simulink model "AGTF30SysDyn_PExPIn"  (R2021b)
settings: Solver=ode4  StartTime=0.0  StopTime=MWS.In.tend  FixedStep=MWS.In.Ts  RelTol=1e-3  EnableMultiTasking=on
model workspace: external: MAT-File (data not in the file)
values from neighbouring files (symbols this model uses):
  MWS = setup_initialize(MWS,startPt,SSsolverSP)    [Setup_Simulation.m]    (also in run_AGTF30e_script.m = Setup_Simulation(inputMethod,MWS.In,filename,Mdl,SSsolverSP,)
undefined symbols (not defined in the file or in its folder): DiscIntNeverNeededParam
libraries: Lib_Solve_ModelSource_TMATS x28, Lib_Cntrl_FirstOrderSensor_TMATS x19, simulink x12, Lib_Cntrl_FirstOrderActuator_TMATS x2, Lib_Cntrl_LimitSelect_TMATS x2, Lib_Solve_OuterLoopIntegrator_TMATS x2, Lib_Cntrl_CorrectedSpeed_TMATS x1, Lib_Solve_IterNRSolverJC_TMATS x1
(part 4 of 6)

== system AGTF30SysDyn_PExPIn/Control System/Wf Controller/Controller/N1cSP Limit Controllers ==
  Prelookup : Inport
  N1 : Inport  Port=2
  N3 : Inport  Port=3
  Ps3 : Inport  Port=4
  T3 : Inport  Port=5
  T4 : Inport  Port=6
  T45 : Inport  Port=7
  N1cCmd : Inport  Port=8
  Mux : Mux  Inputs=7
  N1 Max Controller : Subsystem
  N3 Max Controller : Subsystem
  Ps3 Max Controller : Subsystem
  Ps3 Min Controller : Subsystem
  T3 Max Controller : Subsystem
  T4 Max Controller : Subsystem
  T45 Max Controller : Subsystem
  N1cSP T3 Max : Outport  VectorParamsAs1DForOutWhenUnconnected=off
  N1cSP T4 Max : Outport  Port=2  VectorParamsAs1DForOutWhenUnconnected=off
  N1cSP T45 Max : Outport  Port=3  VectorParamsAs1DForOutWhenUnconnected=off
  N1cSP N1 Max : Outport  Port=4  VectorParamsAs1DForOutWhenUnconnected=off
  N1cSP N3 Max : Outport  Port=5  VectorParamsAs1DForOutWhenUnconnected=off
  N1cSP Ps3 Max : Outport  Port=6  VectorParamsAs1DForOutWhenUnconnected=off
  N1cSP Ps3 Min : Outport  Port=7  VectorParamsAs1DForOutWhenUnconnected=off
  SPs : Outport  Port=8  VectorParamsAs1DForOutWhenUnconnected=off
  wires:
  T3 Max Controller/1(N1cDmd) -> N1cSP T3 Max/1
  T4 Max Controller/1(N1cDmd) -> N1cSP T4 Max/1
  Ps3 Min Controller/1(N1cDmd) -> N1cSP Ps3 Min/1
  N3 Max Controller/1(N1cDmd) -> N1cSP N3 Max/1
  Ps3 Max Controller/1(N1cDmd) -> N1cSP Ps3 Max/1
  T3 Max Controller/2(T3Max_SP) -> Mux/1  "T3Max"
  Mux/1 -> SPs/1
  N1 Max Controller/1(N1cDmd) -> N1cSP N1 Max/1
  N1/1 -> N1 Max Controller/2(N1)
  N3/1 -> N3 Max Controller/2(N3)
  T3/1 -> T3 Max Controller/2(T3)
  T4/1 -> T4 Max Controller/2(T4)
  Ps3/1 -> Ps3 Min Controller/2(Ps3), Ps3 Max Controller/2(Ps3)
  N1cCmd/1 -> T45 Max Controller/3(N1cCmd), Ps3 Min Controller/3(N1cCmd), Ps3 Max Controller/3(N1cCmd), N3 Max Controller/3(N1cCmd), N1 Max Controller/3(N1cCmd), T4 Max Controller/3(N1cCmd), T3 Max Controller/3(N1cCmd)
  T4 Max Controller/2(T4Max_SP) -> Mux/2  "T4Max"
  Ps3 Max Controller/2(Ps3Max_SP) -> Mux/6  "Ps3Max"
  N1 Max Controller/2(N1Max_SP) -> Mux/4  "N1Max"
  N3 Max Controller/2(N3Max_SP) -> Mux/5  "N3Max"
  Ps3 Min Controller/2(Ps3Min_SP) -> Mux/7  "Ps3Min"
  Prelookup/1 -> T45 Max Controller/1(Prelookup), Ps3 Min Controller/1(Prelookup), Ps3 Max Controller/1(Prelookup), N3 Max Controller/1(Prelookup), N1 Max Controller/1(Prelookup), T4 Max Controller/1(Prelookup), T3 Max Controller/1(Prelookup)
  T45/1 -> T45 Max Controller/2(T45)
  T45 Max Controller/2(T4Max_SP) -> Mux/3  "T45Max"
  T45 Max Controller/1(N1cDmd) -> N1cSP T45 Max/1

== system AGTF30SysDyn_PExPIn/Control System/Wf Controller/Controller/N1cSP Limit Select ==
  N1cSPReq : Inport
  Limits : Inport  Port=2
  Limit Selection : Lib_Cntrl_LimitSelect_TMATS/Limit Selection  SelectVec_M=MWS.Cntrl.WfCntrl.N1cSPLim.Type  LimitsEn_M=MWS.Cntrl.WfCntrl.N1cSPLim.En
  N1cSPdmd : Outport  VectorParamsAs1DForOutWhenUnconnected=off
  RegNum : Outport  Port=2  VectorParamsAs1DForOutWhenUnconnected=off
  wires:
  Limit Selection/2 -> RegNum/1
  Limit Selection/1 -> N1cSPdmd/1
  Limits/1 -> Limit Selection/2
  N1cSPReq/1 -> Limit Selection/1

== system AGTF30SysDyn_PExPIn/Control System/Wf Controller/Controller/Nominal Controller ==
  Prelookup : Inport
  N1cManEn : Inport  Port=2
  N1cMan : Inport  Port=3
  N1cSP : Inport  Port=4
  N1c : Inport  Port=5
  Wfcmd : Inport  Port=6
  Bus Selector : BusSelector  OutputSignals=k_PL,f_PL,k_Alt,f_Alt,k_MN,f_MN,k_PwrInLP,f_PwrInLP,k_PwrInHP,f_PwrInHP
  Constant : Constant  Value=MWS.Init.IC.Wf
  Discrete-Time Integrator : DiscreteIntegrator  SampleTime=MWS.In.Ts  ICPrevOutput=DiscIntNeverNeededParam  ICPrevScaledInput=DiscIntNeverNeededParam
  Divide2 : Product  Inputs=**
  Divide3 : Product  Inputs=**
  Gain : Gain  Gain=MWS.Cntrl.WfCntrl.Nom.Kiwp
  Ki Interpolation Using Prelookup : Interpolation_n-D  NumberOfTableDimensions=5  Table=MWS.Cntrl.WfCntrl.Nom.Ki_array  InternalRulePriority=Speed
      settings: InputPortMap=u0,u1,u2,u3,u4,u5,u6,u7,u8,u9
  Kp Interpolation Using Prelookup : Interpolation_n-D  NumberOfTableDimensions=5  Table=MWS.Cntrl.WfCntrl.Nom.Kp_array  InternalRulePriority=Speed
      settings: InputPortMap=u0,u1,u2,u3,u4,u5,u6,u7,u8,u9
  Sum : Sum  Inputs=|+-
  Sum1 : Sum  Inputs=|++
  Sum2 : Sum  Inputs=|-+
  Sum3 : Sum  Inputs=|+-
  Sum4 : Sum  Inputs=|++
  Switch : Switch  Criteria=u2 > Threshold
  Wfdmd : Outport  VectorParamsAs1DForOutWhenUnconnected=off
  N1cErr : Outport  Port=2  VectorParamsAs1DForOutWhenUnconnected=off
  wires:
  Ki Interpolation Using Prelookup/1 -> Divide2/1  "Ki"
  N1c/1 -> Sum/2
  Divide2/1 -> Discrete-Time Integrator/1
  Sum/1 -> N1cErr/1, [Error]
  Constant/1 -> Sum4/2
  Discrete-Time Integrator/1 -> Sum1/2
  Kp Interpolation Using Prelookup/1 -> Divide3/1  "Kp"
  Sum1/1 -> Sum4/1
  [Error] -> Divide3/2
  Divide3/1 -> Sum1/1
  Sum2/1 -> Gain/1
  Gain/1 -> Sum3/2
  Sum4/1 -> Sum2/2, Wfdmd/1
  [Error] -> Sum3/1
  Wfcmd/1 -> Sum2/1
  Sum3/1 -> Divide2/2
  Prelookup/1 -> Bus Selector/1
  Bus Selector/1 -> Ki Interpolation Using Prelookup/1, Kp Interpolation Using Prelookup/1  "<k_PL>"
  Bus Selector/2 -> Ki Interpolation Using Prelookup/2, Kp Interpolation Using Prelookup/2  "<f_PL>"
  Bus Selector/3 -> Ki Interpolation Using Prelookup/3, Kp Interpolation Using Prelookup/3  "<k_Alt>"
  Bus Selector/4 -> Ki Interpolation Using Prelookup/4, Kp Interpolation Using Prelookup/4  "<f_Alt>"
  Bus Selector/5 -> Ki Interpolation Using Prelookup/5, Kp Interpolation Using Prelookup/5  "<k_MN>"
  Bus Selector/6 -> Ki Interpolation Using Prelookup/6, Kp Interpolation Using Prelookup/6  "<f_MN>"
  Bus Selector/10 -> Ki Interpolation Using Prelookup/10, Kp Interpolation Using Prelookup/10  "<f_PwrInHP>"
  Bus Selector/7 -> Ki Interpolation Using Prelookup/7, Kp Interpolation Using Prelookup/7  "<k_PwrInLP>"
  Bus Selector/8 -> Ki Interpolation Using Prelookup/8, Kp Interpolation Using Prelookup/8  "<f_PwrInLP>"
  Bus Selector/9 -> Ki Interpolation Using Prelookup/9, Kp Interpolation Using Prelookup/9  "<k_PwrInHP>"
  Switch/1 -> Sum/1
  N1cSP/1 -> Switch/3  "N1cSP"
  N1cMan/1 -> Switch/1  "N1cSP"
  N1cManEn/1 -> Switch/2

== system AGTF30SysDyn_PExPIn/Control System/Wf Controller/Controller/Nominal Set-Point Determination ==
  Prelookup : Inport
  Bus Selector : BusSelector  OutputSignals=k_PL_Targ,f_PL_Targ,k_Alt,f_Alt,k_MN,f_MN,k_PwrInLP,f_PwrInLP,k_PwrInHP,f_PwrInHP
  NcFanSP Interpolation Using Prelookup : Interpolation_n-D  NumberOfTableDimensions=5  Table=MWS.Cntrl.WfCntrl.Sched.N1cSP.N1cSP_array  InternalRulePriority=Speed
      settings: InputPortMap=u0,u1,u2,u3,u4,u5,u6,u7,u8,u9
  N1cSP : Outport  VectorParamsAs1DForOutWhenUnconnected=off
  wires:
  Prelookup/1 -> Bus Selector/1
  Bus Selector/1 -> NcFanSP Interpolation Using Prelookup/1  "<k_PL_Targ>"
  Bus Selector/2 -> NcFanSP Interpolation Using Prelookup/2  "<f_PL_Targ>"
  Bus Selector/3 -> NcFanSP Interpolation Using Prelookup/3  "<k_Alt>"
  Bus Selector/4 -> NcFanSP Interpolation Using Prelookup/4  "<f_Alt>"
  Bus Selector/5 -> NcFanSP Interpolation Using Prelookup/5  "<k_MN>"
  Bus Selector/6 -> NcFanSP Interpolation Using Prelookup/6  "<f_MN>"
  Bus Selector/7 -> NcFanSP Interpolation Using Prelookup/7  "<k_PwrInLP>"
  Bus Selector/8 -> NcFanSP Interpolation Using Prelookup/8  "<f_PwrInLP>"
  Bus Selector/9 -> NcFanSP Interpolation Using Prelookup/9  "<k_PwrInHP>"
  Bus Selector/10 -> NcFanSP Interpolation Using Prelookup/10  "<f_PwrInHP>"
  NcFanSP Interpolation Using Prelookup/1 -> N1cSP/1

== system AGTF30SysDyn_PExPIn/Control System/Wf Controller/Controller/Set-Points ==
  Nominal SP : Inport
  N1cSP Limit SPs : Inport  Port=2
  Wf Limit SPs : Inport  Port=3
  Bus Creator : BusCreator  Inputs=3
  Bus Creator1 : BusCreator  Inputs=7
  Bus Creator2 : BusCreator  Inputs=3
  Demux : Demux  Outputs=7
  Demux1 : Demux  Outputs=3
  SPs : Outport  VectorParamsAs1DForOutWhenUnconnected=off
  wires:
  Nominal SP/1 -> Bus Creator/1  "N1c"
  N1cSP Limit SPs/1 -> Demux/1
  Bus Creator/1 -> SPs/1
  Demux/1 -> Bus Creator1/1  "T3Max"
  Demux/2 -> Bus Creator1/2  "T4Max"
  Demux/3 -> Bus Creator1/3  "T45Max"
  Demux/4 -> Bus Creator1/4  "N1Max"
  Demux/5 -> Bus Creator1/5  "N3Max"
  Demux/6 -> Bus Creator1/6  "Ps3Max"
  Demux/7 -> Bus Creator1/7  "Ps3Min"
  Bus Creator1/1 -> Bus Creator/2  "N1cSPLims"
  Bus Creator2/1 -> Bus Creator/3  "WfLims"
  Demux1/1 -> Bus Creator2/1  "Accel"
  Demux1/2 -> Bus Creator2/2  "Decel"
  Demux1/3 -> Bus Creator2/3  "WfMin"
  Wf Limit SPs/1 -> Demux1/1

== system AGTF30SysDyn_PExPIn/Control System/Wf Controller/Controller/Wf Limit Controllers ==
  Alt : Inport
  MN : Inport  Port=2
  Wfmin : Inport  Port=3
  Wfmax : Inport  Port=4
  Wfcmd : Inport  Port=5
  phiEPT : Inport  Port=6
  phiBoost : Inport  Port=7
  N1cN : Inport  Port=8
  ps3 : Inport  Port=9
  Accel Controller : Subsystem
  Decel Controller : Subsystem
  Gain : Gain  Gain=0.95; %0.95
  Mux : Mux  Inputs=3
  Wf Accel : Outport  VectorParamsAs1DForOutWhenUnconnected=off
  Wf Decel : Outport  Port=2  VectorParamsAs1DForOutWhenUnconnected=off
  Wf Min : Outport  Port=3  VectorParamsAs1DForOutWhenUnconnected=off
  SPs : Outport  Port=4  VectorParamsAs1DForOutWhenUnconnected=off
  wires:
  Gain/1 -> Mux/3, Wf Min/1  "WfMin"
  Alt/1 -> Decel Controller/1(Alt), Accel Controller/1(Alt)
  Wfmax/1 -> Accel Controller/6(Wfmax)
  Decel Controller/2(WfminDecel_SP) -> Mux/2  "WfMinDecel"
  Accel Controller/2(WfmaxAccel_SP) -> Mux/1  "WfMaxAccel"
  Wfcmd/1 -> Accel Controller/7(Wfcmd), Decel Controller/7(Wf)
  Wfmin/1 -> Gain/1, Decel Controller/6(Wfmin)
  Decel Controller/1(Wfdmd) -> Wf Decel/1
  Accel Controller/1(Wfdmd) -> Wf Accel/1
  Mux/1 -> SPs/1
  MN/1 -> Decel Controller/2(MN), Accel Controller/2(MN)
  phiEPT/1 -> Decel Controller/4(phiEPT), Accel Controller/4(phiEPT)
  phiBoost/1 -> Decel Controller/5(phiBoost), Accel Controller/5(phiBoost)
  ps3/1 -> Accel Controller/8(ps3), Decel Controller/8(ps3)
  N1cN/1 -> Decel Controller/3(N1cN), Accel Controller/3(N1cN)

== system AGTF30SysDyn_PExPIn/Control System/Wf Controller/Controller/Wf Limit Select ==
  WfReq : Inport
  Limits : Inport  Port=2
  Limit Selection : Lib_Cntrl_LimitSelect_TMATS/Limit Selection  SelectVec_M=MWS.Cntrl.WfCntrl.WfLim.Type  LimitsEn_M=MWS.Cntrl.WfCntrl.WfLim.En
  Wfdmd : Outport  VectorParamsAs1DForOutWhenUnconnected=off
  RegNum : Outport  Port=2  VectorParamsAs1DForOutWhenUnconnected=off
  wires:
  WfReq/1 -> Limit Selection/1
  Limits/1 -> Limit Selection/2
  Limit Selection/1 -> Wfdmd/1
  Limit Selection/2 -> RegNum/1

== system AGTF30SysDyn_PExPIn/Control System/Electric Machine Controllers/VEATE EM Controllers/Base Power/Base Power - Boost and PEx ==
  note: 1: HP-Sun, LP-Ring, Coupling-Carrier
      | 2: HP-Sun, LP-Carrier, Coupling-Ring
      | 3: HP-Ring, LP-Sun, Coupling-Carrier
      | 4: HP-Ring, LP-Carrier, Coupling-Sun
      | 5: HP-Carrier, LP-Sun, Coupling-Ring
      | 6: HP-Carrier, LP-Ring, Coupling-Sun
  PwrL_Base : Inport
  PwrH_Base : Inport  Port=2
  NS : Inport  Port=3
  NR : Inport  Port=4
  NC : Inport  Port=5
  Boost PEx - HC LR CS : Subsystem
  Boost PEx - HC LS CR : Subsystem
  "Boost PEx - HR LC CS " : Subsystem
  Boost PEx - HR LS CC : Subsystem
  Boost PEx - HS LC CR : Subsystem
  Boost PEx - HS LR CC : Subsystem
  Constant1 : Constant  Value=MWS.In.Options.PGBConfig
  Multiport Switch4 : MultiPortSwitch  Inputs=6
  Mux{1..6} (6 alike) : Mux
  Pem : Outport
  wires:
  Boost PEx - HC LS CR/1(PemS_Base) -> Mux5/1
  Boost PEx - HC LR CS/1(PemS_Base) -> Mux6/1
  NS/1 -> Boost PEx - HC LR CS/3(NS), Boost PEx - HC LS CR/3(NS), "Boost PEx - HR LC CS "/3(NS), Boost PEx - HR LS CC/3(NS), Boost PEx - HS LC CR/3(NS), Boost PEx - HS LR CC/3(NS)
  Boost PEx - HC LS CR/4(PemP_Base) -> Mux5/4
  Boost PEx - HC LR CS/2(PemR_Base) -> Mux6/2
  Boost PEx - HC LR CS/3(PemC_Base) -> Mux6/3
  PwrH_Base/1 -> Boost PEx - HC LR CS/2(PwrH_Base), Boost PEx - HC LS CR/2(PwrH_Base), "Boost PEx - HR LC CS "/2(PwrH_Base), Boost PEx - HR LS CC/2(PwrH_Base), Boost PEx - HS LC CR/2(PwrH_Base), Boost PEx - HS LR CC/2(PwrH_Base)
  NR/1 -> Boost PEx - HC LR CS/4(NR), Boost PEx - HC LS CR/4(NR), "Boost PEx - HR LC CS "/4(NR), Boost PEx - HR LS CC/4(NR), Boost PEx - HS LC CR/4(NR), Boost PEx - HS LR CC/4(NR)
  Mux4/1 -> [Pem_HRLCCS]
  Mux6/1 -> [Pem_HCLRCS]
  Mux2/1 -> [Pem_HSLCCR]
  Boost PEx - HC LS CR/3(PemC_Base) -> Mux5/3
  PwrL_Base/1 -> Boost PEx - HC LR CS/1(PwrL_Base), Boost PEx - HC LS CR/1(PwrL_Base), "Boost PEx - HR LC CS "/1(PwrL_Base), Boost PEx - HR LS CC/1(PwrL_Base), Boost PEx - HS LC CR/1(PwrL_Base), Boost PEx - HS LR CC/1(PwrL_Base)
  Boost PEx - HS LC CR/3(PemC_Base) -> Mux2/3
  Boost PEx - HS LR CC/2(PemR_Base) -> Mux1/2
  Boost PEx - HR LS CC/1(PemS_Base) -> Mux3/1
  Mux1/1 -> [Pem_HSLRCC]
  Boost PEx - HS LR CC/4(PemP_Base) -> Mux1/4
  Constant1/1 -> Multiport Switch4/1
  NC/1 -> Boost PEx - HC LR CS/5(NC), Boost PEx - HC LS CR/5(NC), "Boost PEx - HR LC CS "/5(NC), Boost PEx - HR LS CC/5(NC), Boost PEx - HS LC CR/5(NC), Boost PEx - HS LR CC/5(NC)
  [Pem_HSLCCR] -> Multiport Switch4/3
  Boost PEx - HC LR CS/4(PemP_Base) -> Mux6/4
  [Pem_HRLCCS] -> Multiport Switch4/5
  Boost PEx - HS LC CR/1(PemS_Base) -> Mux2/1
  Boost PEx - HC LS CR/2(PemR_Base) -> Mux5/2
  Boost PEx - HS LC CR/2(PemR_Base) -> Mux2/2
  Boost PEx - HS LC CR/4(PemP_Base) -> Mux2/4
  Boost PEx - HR LS CC/2(PemR_Base) -> Mux3/2
  Mux5/1 -> [Pem_HCLSCR]
  "Boost PEx - HR LC CS "/2(PemR_Base) -> Mux4/2
  Boost PEx - HR LS CC/4(PemP_Base) -> Mux3/4
  [Pem_HCLSCR] -> Multiport Switch4/6
  Boost PEx - HR LS CC/3(PemC_Base) -> Mux3/3
  "Boost PEx - HR LC CS "/3(PemC_Base) -> Mux4/3
  [Pem_HSLRCC] -> Multiport Switch4/2
  Mux3/1 -> [Pem_HRLSCC]
  "Boost PEx - HR LC CS "/4(PemP_Base) -> Mux4/4
  "Boost PEx - HR LC CS "/1(PemS_Base) -> Mux4/1
  Boost PEx - HS LR CC/3(PemC_Base) -> Mux1/3
  Boost PEx - HS LR CC/1(PemS_Base) -> Mux1/1
  [Pem_HCLRCS] -> Multiport Switch4/7
  [Pem_HRLSCC] -> Multiport Switch4/4
  Multiport Switch4/1 -> Pem/1

== system AGTF30SysDyn_PExPIn/Control System/Electric Machine Controllers/VEATE EM Controllers/Base Power/Base Power - Standard ==
  note: 1: HP-Sun, LP-Ring, Coupling-Carrier
      | 2: HP-Sun, LP-Carrier, Coupling-Ring
      | 3: HP-Ring, LP-Sun, Coupling-Carrier
      | 4: HP-Ring, LP-Carrier, Coupling-Sun
      | 5: HP-Carrier, LP-Sun, Coupling-Ring
      | 6: HP-Carrier, LP-Ring, Coupling-Sun
  PwrH_Base : Inport
  NS : Inport  Port=2
  NR : Inport  Port=3
  NC : Inport  Port=4
  Constant1 : Constant  Value=MWS.In.Options.PGBConfig
  Multiport Switch4 : MultiPortSwitch  Inputs=6
  Mux1 : Mux
  Mux2 : Mux
  Mux3 : Mux
  Standard - HC : Subsystem
  Standard - HR : Subsystem
  Standard - HS : Subsystem
  Pem : Outport
  wires:
  Multiport Switch4/1 -> Pem/1
  Standard - HS/1(PemS_Base) -> Mux1/1
  Standard - HS/3(PemC_Base) -> Mux1/3
  [Pem_HS] -> Multiport Switch4/3, Multiport Switch4/2
  Constant1/1 -> Multiport Switch4/1
  Standard - HS/4(PemP_Base) -> Mux1/4
  Mux1/1 -> [Pem_HS]
  Standard - HS/2(PemR_Base) -> Mux1/2
  PwrH_Base/1 -> Standard - HC/1(PwrH_Base), Standard - HR/1(PwrH_Base), Standard - HS/1(PwrH_Base)
  NS/1 -> Standard - HS/2(NS)
  [Pem_HR] -> Multiport Switch4/5, Multiport Switch4/4
  [Pem_HC] -> Multiport Switch4/7, Multiport Switch4/6
  Standard - HR/2(PemR_Base) -> Mux2/2
  Standard - HR/4(PemP_Base) -> Mux2/4
  Standard - HR/3(PemC_Base) -> Mux2/3
  Standard - HR/1(PemS_Base) -> Mux2/1
  Mux2/1 -> [Pem_HR]
  NR/1 -> Standard - HR/2(NR)
  Mux3/1 -> [Pem_HC]
  Standard - HC/1(PemS_Base) -> Mux3/1
  Standard - HC/3(PemC_Base) -> Mux3/3
  Standard - HC/4(PemP_Base) -> Mux3/4
  Standard - HC/2(PemR_Base) -> Mux3/2
  NC/1 -> Standard - HC/2(NS)

== system AGTF30SysDyn_PExPIn/Control System/Electric Machine Controllers/VEATE EM Controllers/Base Power/Subsystem ==
  PwrLoad : Inport
  Demux : Demux  Outputs=[3 1]
  Gain1 : Gain  Gain=MWS.Shaft.PGB.Planet.nP
  Mux : Mux  Inputs=2
  PwrLoadTot : Outport
  wires:
  Gain1/1 -> Mux/2
  PwrLoad/1 -> Demux/1
  Demux/2 -> Gain1/1
  Demux/1 -> Mux/1
  Mux/1 -> PwrLoadTot/1

== system AGTF30SysDyn_PExPIn/Control System/Electric Machine Controllers/VEATE EM Controllers/TEEM Power/TEEM Power ==
  note: NEED TO MODIFY THIS!!!!!!!!!!!!!!!!!!!!!!!!!!!!!!!!!!!!!!
  note: 1: HP-Sun, LP-Ring, Coupling-Carrier
      | 2: HP-Sun, LP-Carrier, Coupling-Ring
      | 3: HP-Ring, LP-Sun, Coupling-Carrier
      | 4: HP-Ring, LP-Carrier, Coupling-Sun
      | 5: HP-Carrier, LP-Sun, Coupling-Ring
      | 6: HP-Carrier, LP-Ring, Coupling-Sun
  PwrInAccel_TEEM : Inport
  PwrXDecel_TEEM : Inport  Port=2
  NS : Inport  Port=3
  NR : Inport  Port=4
  NC : Inport  Port=5
  Constant1 : Constant  Value=MWS.In.Options.PGBConfig
  Multiport Switch4 : MultiPortSwitch  Inputs=6
  Mux{1..6} (6 alike) : Mux
  Sum : Sum  Inputs=|++
  TEEM - HC LR CS : Subsystem
  TEEM - HC LS CR : Subsystem
  "TEEM - HR LC CS " : Subsystem
  TEEM - HR LS CC : Subsystem
  TEEM - HS LC CR : Subsystem
  TEEM- HS LR CC : Subsystem
  Pem : Outport
  wires:
  Multiport Switch4/1 -> Pem/1
  [Pem_HRLSCC] -> Multiport Switch4/4
  [Pem_HCLRCS] -> Multiport Switch4/7
  TEEM- HS LR CC/1(PemS_TEEM) -> Mux1/1
  TEEM- HS LR CC/3(PemC_TEEM) -> Mux1/3
  "TEEM - HR LC CS "/1(PemS_TEEM) -> Mux4/1
  "TEEM - HR LC CS "/4(PemP_TEEM) -> Mux4/4
  Mux3/1 -> [Pem_HRLSCC]
  [Pem_HSLRCC] -> Multiport Switch4/2
  "TEEM - HR LC CS "/3(PemC_TEEM) -> Mux4/3
  TEEM - HR LS CC/3(PemC_TEEM) -> Mux3/3
  [Pem_HCLSCR] -> Multiport Switch4/6
  TEEM - HR LS CC/4(PemP_TEEM) -> Mux3/4
  "TEEM - HR LC CS "/2(PemR_TEEM) -> Mux4/2
  Mux5/1 -> [Pem_HCLSCR]
  TEEM - HR LS CC/2(PemR_TEEM) -> Mux3/2
  TEEM - HS LC CR/4(PemP_TEEM) -> Mux2/4
  TEEM - HS LC CR/2(PemR_TEEM) -> Mux2/2
  TEEM - HC LS CR/2(PemR_TEEM) -> Mux5/2
  TEEM - HS LC CR/1(PemS_TEEM) -> Mux2/1
  [Pem_HRLCCS] -> Multiport Switch4/5
  TEEM - HC LR CS/4(PemP_TEEM) -> Mux6/4
  [Pem_HSLCCR] -> Multiport Switch4/3
  NC/1 -> TEEM - HC LR CS/3(NC), TEEM - HC LS CR/3(NC), TEEM - HR LS CC/3(NC), TEEM- HS LR CC/3(NC)
  Constant1/1 -> Multiport Switch4/1
  TEEM- HS LR CC/4(PemP_TEEM) -> Mux1/4
  Mux1/1 -> [Pem_HSLRCC]
  TEEM - HR LS CC/1(PemS_TEEM) -> Mux3/1
  TEEM- HS LR CC/2(PemR_TEEM) -> Mux1/2
  TEEM - HS LC CR/3(PemC_TEEM) -> Mux2/3
  TEEM - HC LS CR/3(PemC_TEEM) -> Mux5/3
  Mux2/1 -> [Pem_HSLCCR]
  Mux6/1 -> [Pem_HCLRCS]
  Mux4/1 -> [Pem_HRLCCS]
  NR/1 -> TEEM - HC LS CR/2(NR), "TEEM - HR LC CS "/3(NR), TEEM - HR LS CC/2(NR), TEEM - HS LC CR/3(NR)
  TEEM - HC LR CS/3(PemC_TEEM) -> Mux6/3
  TEEM - HC LR CS/2(PemR_TEEM) -> Mux6/2
  TEEM - HC LS CR/4(PemP_TEEM) -> Mux5/4
  NS/1 -> TEEM - HC LR CS/2(NS), "TEEM - HR LC CS "/2(NS), TEEM - HS LC CR/2(NS), TEEM- HS LR CC/2(NS)
  TEEM - HC LR CS/1(PemS_TEEM) -> Mux6/1
  TEEM - HC LS CR/1(PemS_TEEM) -> Mux5/1
  PwrInAccel_TEEM/1 -> Sum/1
  PwrXDecel_TEEM/1 -> Sum/2
  Sum/1 -> [Pwr_TEEM]
  [Pwr_TEEM] -> TEEM - HC LR CS/1(Pwr_TEEM), TEEM - HC LS CR/1(Pwr_TEEM), "TEEM - HR LC CS "/1(Pwr_TEEM), TEEM - HR LS CC/1(Pwr_TEEM), TEEM - HS LC CR/1(Pwr_TEEM), TEEM- HS LR CC/1(Pwr_TEEM)

== system AGTF30SysDyn_PExPIn/Control System/Scheduling/Steady State EM Power - MaxMin/HP and LP Pwr Calc/Gearbox Speeds ==
  k_Alt : Inport
  f_Alt : Inport  Port=2
  k_MN : Inport  Port=3
  f_MN : Inport  Port=4
  PwrBase_LP : Inport  Port=5
  PwrBase_HP : Inport  Port=6
  PwrEPT_LPg : Inport  Port=7
  PwrEPT_HPg : Inport  Port=8
  Constant35 : Constant  Value=[[0:1:length(MWS.Cntrl.SPSched.PL_vec)-2],length(MWS.Cntrl.SPSched.PL_vec)-2]
  Constant36 : Constant  Value=[zeros(1,length(MWS.Cntrl.SPSched.PL_vec)-1),1]
  Mux12 : Mux  Inputs=2
  N2 Interpolation Using Prelookup : Interpolation_n-D  NumberOfTableDimensions=5  Table=MWS.Cntrl.Sched.N2.N2_array  InternalRulePriority=Speed
      settings: InputPortMap=u0,u1,u2,u3,u4,u5,u6,u7,u8,u9
  N2min Lookup Table Dynamic : simulink/Lookup Tables/Lookup Table Dynamic  LookUpMeth=Interpolation-Use End Values  OutDataType=fixdt('double')  OutScaling=[]  OutputDataTypeScalingMode=Specify via dialog  OutDataTypeStr=double  DoSatur=off
  N3 Interpolation Using Prelookup : Interpolation_n-D  NumberOfTableDimensions=5  Table=MWS.Cntrl.Sched.N3.N3_array  InternalRulePriority=Speed
      settings: InputPortMap=u0,u1,u2,u3,u4,u5,u6,u7,u8,u9
  N3min Lookup Table Dynamic : simulink/Lookup Tables/Lookup Table Dynamic  LookUpMeth=Interpolation-Use End Values  OutDataType=fixdt('double')  OutScaling=[]  OutputDataTypeScalingMode=Specify via dialog  OutDataTypeStr=double  DoSatur=off
  Ps3 Interpolation Using Prelookup : Interpolation_n-D  NumberOfTableDimensions=5  Table=MWS.Cntrl.Sched.Ps3.Ps3_array  InternalRulePriority=Speed
      settings: InputPortMap=u0,u1,u2,u3,u4,u5,u6,u7,u8,u9
  Ps3min Interpolation Using Prelookup : Interpolation_n-D  Table=MWS.Cntrl.Sched.Ps3Min.Ps3Min_array  InterpMethod=Linear Lagrange  InternalRulePriority=Speed
  PwrInHP Prelookup : PreLookup  BreakpointsData=MWS.Cntrl.SPSched.PwrInHP_vec  IndexSearchMethod=Linear search  BeginIndexSearchUsingPreviousIndexResult=on  ExtrapMethod=Linear
  PwrInLP Prelookup : PreLookup  BreakpointsData=MWS.Cntrl.SPSched.PwrInLP_vec  IndexSearchMethod=Linear search  BeginIndexSearchUsingPreviousIndexResult=on  ExtrapMethod=Linear
  Spool to PGB speeds : Subsystem
  Sum : Sum  Inputs=|++
  Sum1 : Sum  Inputs=|++
  NPGB : Outport
  wires:
  [N3vec] -> N3min Lookup Table Dynamic/3
  Spool to PGB speeds/1(NPGB) -> NPGB/1
  [f_PwrInHP] -> N2 Interpolation Using Prelookup/10, N3 Interpolation Using Prelookup/10, Ps3 Interpolation Using Prelookup/10
  [f_PwrInLP] -> N2 Interpolation Using Prelookup/8, N3 Interpolation Using Prelookup/8, Ps3 Interpolation Using Prelookup/8
  [k_PwrInHP] -> N2 Interpolation Using Prelookup/9, N3 Interpolation Using Prelookup/9, Ps3 Interpolation Using Prelookup/9
  N2 Interpolation Using Prelookup/1 -> [N2vec]
  k_Alt/1 -> N2 Interpolation Using Prelookup/3, N3 Interpolation Using Prelookup/3, Ps3 Interpolation Using Prelookup/3, Ps3min Interpolation Using Prelookup/1
  PwrInLP Prelookup/1 -> [k_PwrInLP]  "k_PwrInHPMn"
  N3min Lookup Table Dynamic/1 -> Mux12/2  "N3min"
  f_MN/1 -> N2 Interpolation Using Prelookup/6, N3 Interpolation Using Prelookup/6, Ps3 Interpolation Using Prelookup/6, Ps3min Interpolation Using Prelookup/4
  PwrEPT_LPg/1 -> Sum/2
  k_MN/1 -> N2 Interpolation Using Prelookup/5, N3 Interpolation Using Prelookup/5, Ps3 Interpolation Using Prelookup/5, Ps3min Interpolation Using Prelookup/3
  Constant35/1 -> N3 Interpolation Using Prelookup/1, N2 Interpolation Using Prelookup/1, Ps3 Interpolation Using Prelookup/1
  PwrInHP Prelookup/1 -> [k_PwrInHP]  "k_PwrInHPMn"
  f_Alt/1 -> N2 Interpolation Using Prelookup/4, N3 Interpolation Using Prelookup/4, Ps3 Interpolation Using Prelookup/4, Ps3min Interpolation Using Prelookup/2
  [k_PwrInLP] -> N2 Interpolation Using Prelookup/7, N3 Interpolation Using Prelookup/7, Ps3 Interpolation Using Prelookup/7
  [Ps3vec] -> N2min Lookup Table Dynamic/2
  Sum1/1 -> PwrInHP Prelookup/1
  [Ps3vec] -> N3min Lookup Table Dynamic/2
  Constant36/1 -> N3 Interpolation Using Prelookup/2, N2 Interpolation Using Prelookup/2, Ps3 Interpolation Using Prelookup/2
  PwrBase_HP/1 -> Sum1/1
  PwrInHP Prelookup/2 -> [f_PwrInHP]  "f_PwrInHPMx"
  [Ps3min] -> N3min Lookup Table Dynamic/1
  Ps3 Interpolation Using Prelookup/1 -> [Ps3vec]
  [N2vec] -> N2min Lookup Table Dynamic/3
  Ps3min Interpolation Using Prelookup/1 -> [Ps3min]
  Sum/1 -> PwrInLP Prelookup/1
  PwrEPT_HPg/1 -> Sum1/2
  [Ps3min] -> N2min Lookup Table Dynamic/1
  N3 Interpolation Using Prelookup/1 -> [N3vec]
  PwrInLP Prelookup/2 -> [f_PwrInLP]  "f_PwrInHPMx"
  N2min Lookup Table Dynamic/1 -> Mux12/1  "N2min"
  Mux12/1 -> Spool to PGB speeds/1(N)
  PwrBase_LP/1 -> Sum/1

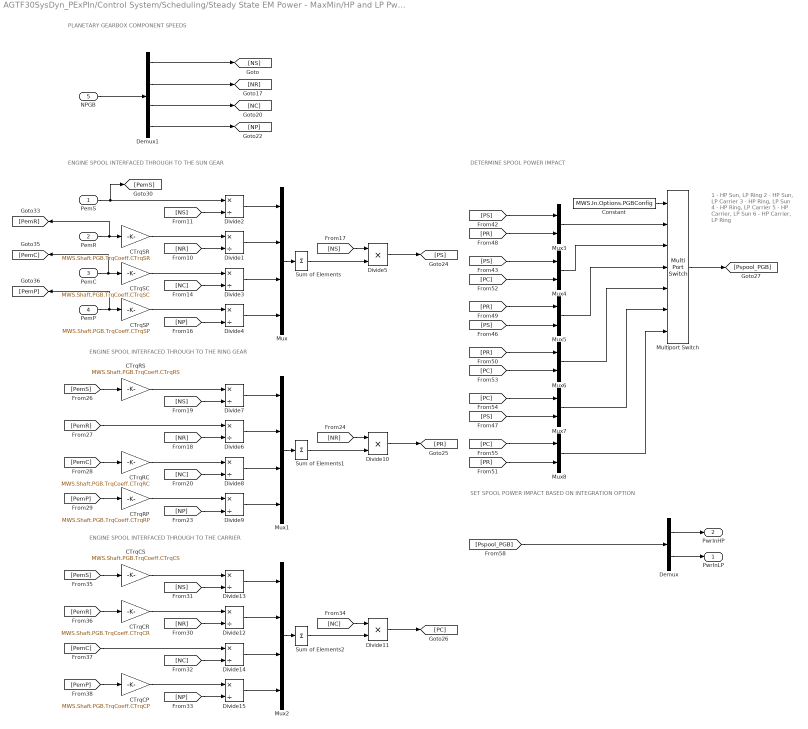
== system AGTF30SysDyn_PExPIn/Control System/Scheduling/Steady State EM Power - MaxMin/HP and LP Pwr Calc/Spool Power Impact ==
  note: 1 - HP Sun, LP Ring
      | 2 - HP Sun, LP Carrier
      | 3 - HP Ring, LP Sun
      | 4 - HP Ring, LP Carrier
      | 5 - HP Carrier, LP Sun
      | 6 - HP Carrier, LP Ring
  note: ENGINE SPOOL INTERFACED THROUGH TO THE SUN GEAR
  note: ENGINE SPOOL INTERFACED THROUGH TO THE RING GEAR
  note: ENGINE SPOOL INTERFACED THROUGH TO THE CARRIER
  note: DETERMINE SPOOL POWER IMPACT
  note: SET SPOOL POWER IMPACT BASED ON INTEGRATION OPTION
  note: PLANETARY GEARBOX COMPONENT SPEEDS
  PemS : Inport
  PemR : Inport  Port=2
  PemC : Inport  Port=3
  PemP : Inport  Port=4
  NPGB : Inport  Port=5
  CTrqCP : Gain  Gain=MWS.Shaft.PGB.TrqCoeff.CTrqCP
  CTrqCR : Gain  Gain=MWS.Shaft.PGB.TrqCoeff.CTrqCR
  CTrqCS : Gain  Gain=MWS.Shaft.PGB.TrqCoeff.CTrqCS
  CTrqRC : Gain  Gain=MWS.Shaft.PGB.TrqCoeff.CTrqRC
  CTrqRP : Gain  Gain=MWS.Shaft.PGB.TrqCoeff.CTrqRP
  CTrqRS : Gain  Gain=MWS.Shaft.PGB.TrqCoeff.CTrqRS
  CTrqSC : Gain  Gain=MWS.Shaft.PGB.TrqCoeff.CTrqSC
  CTrqSP : Gain  Gain=MWS.Shaft.PGB.TrqCoeff.CTrqSP
  CTrqSR : Gain  Gain=MWS.Shaft.PGB.TrqCoeff.CTrqSR
  Constant : Constant  Value=MWS.In.Options.PGBConfig
  Demux : Demux  Outputs=2
  Demux1 : Demux
  Divide{1..4,6..9,12..15} (12 alike) : Product  Inputs=*/
  Divide10 : Product  Inputs=**
  Divide11 : Product  Inputs=**
  Divide5 : Product  Inputs=**
  Multiport Switch : MultiPortSwitch  Inputs=6
  Mux : Mux
  Mux1 : Mux
  Mux2 : Mux
  Mux{3..8} (6 alike) : Mux  Inputs=2
  Sum of Elements : Sum  Inputs=+
  Sum of Elements1 : Sum  Inputs=+
  Sum of Elements2 : Sum  Inputs=+
  PwrInLP : Outport
  PwrInHP : Outport  Port=2
  wires:
  [PemP] -> CTrqRP/1
  CTrqRC/1 -> Divide8/1
  [NP] -> Divide4/2
  CTrqRP/1 -> Divide9/1
  [PemS] -> CTrqCS/1
  Mux8/1 -> Multiport Switch/7
  [NC] -> Divide14/2
  Mux5/1 -> Multiport Switch/4
  [PR] -> Mux5/1
  [NP] -> Divide15/2
  CTrqCS/1 -> Divide13/1
  CTrqCP/1 -> Divide15/1
  [PR] -> Mux3/2
  [PC] -> Mux8/1
  CTrqRS/1 -> Divide7/1
  Divide4/1 -> Mux/4
  [PS] -> Mux5/2
  [Pspool_PGB] -> Demux/1
  [NS] -> Divide7/2
  [PR] -> Mux8/2
  Divide11/1 -> [PC]
  Divide7/1 -> Mux1/1
  CTrqSR/1 -> Divide1/1
  Divide14/1 -> Mux2/3
  [PemC] -> Divide14/1
  [PemC] -> CTrqRC/1
  Mux4/1 -> Multiport Switch/3
  [PC] -> Mux4/2
  [NP] -> Divide9/2
  CTrqSC/1 -> Divide3/1
  Divide2/1 -> Mux/1
  Mux2/1 -> Sum of Elements2/1
  PemR/1 -> [PemR], CTrqSR/1
  [NR] -> Divide12/2
  Divide15/1 -> Mux2/4
  Divide8/1 -> Mux1/3
  [NS] -> Divide2/2
  [PC] -> Mux6/2
  Constant/1 -> Multiport Switch/1
  [PemP] -> CTrqCP/1
  Divide10/1 -> [PR]
  [NC] -> Divide11/1
  Divide3/1 -> Mux/3
  [NS] -> Divide5/1
  Divide13/1 -> Mux2/1
  [NS] -> Divide13/2
  [NR] -> Divide1/2
  Mux6/1 -> Multiport Switch/5
  Divide5/1 -> [PS]
  Divide12/1 -> Mux2/2
  PemP/1 -> [PemP], CTrqSP/1
  [PS] -> Mux3/1
  [NR] -> Divide10/1
  [PR] -> Mux6/1
  PemS/1 -> [PemS], Divide2/1
  [PemS] -> CTrqRS/1
  [NC] -> Divide3/2
  CTrqSP/1 -> Divide4/1
  Mux7/1 -> Multiport Switch/6
  CTrqCR/1 -> Divide12/1
  Divide1/1 -> Mux/2
  [PemR] -> CTrqCR/1
  PemC/1 -> [PemC], CTrqSC/1
  [PC] -> Mux7/1
  [PS] -> Mux7/2
  [PS] -> Mux4/1
  Multiport Switch/1 -> [Pspool_PGB]
  [PemR] -> Divide6/1
  Mux3/1 -> Multiport Switch/2
  [NC] -> Divide8/2
  Divide9/1 -> Mux1/4
  Mux1/1 -> Sum of Elements1/1
  Divide6/1 -> Mux1/2
  [NR] -> Divide6/2
  Mux/1 -> Sum of Elements/1
  Demux/1 -> PwrInHP/1
  Demux/2 -> PwrInLP/1
  NPGB/1 -> Demux1/1
  Demux1/1 -> [NS]
  Demux1/2 -> [NR]
  Demux1/3 -> [NC]
  Demux1/4 -> [NP]
  Sum of Elements/1 -> Divide5/2
  Sum of Elements1/1 -> Divide10/2
  Sum of Elements2/1 -> Divide11/2

== system AGTF30SysDyn_PExPIn/Control System/Wf Controller/Controller/N1cSP Limit Controllers/N1 Max Controller ==
  Prelookup : Inport
  N1 : Inport  Port=2
  N1cCmd : Inport  Port=3
  Bus Selector : BusSelector  OutputSignals=k_Alt,f_Alt,k_MN,f_MN,k_PwrInLP,f_PwrInLP,k_PwrInHP,f_PwrInHP
  Constant : Constant  Value=MWS.Init.IC.N1c
  Constant1 : Constant  Value=MWS.Cntrl.WfCntrl.N1Max.SP
  Discrete-Time Integrator : DiscreteIntegrator  SampleTime=MWS.In.Ts  ICPrevOutput=DiscIntNeverNeededParam  ICPrevScaledInput=DiscIntNeverNeededParam
  Divide2 : Product  Inputs=**
  Divide3 : Product  Inputs=**
  Gain : Gain  Gain=MWS.Cntrl.WfCntrl.N1Max.Kiwp
  Ki Interpolation Using Prelookup : Interpolation_n-D  NumberOfTableDimensions=4  Table=MWS.Cntrl.WfCntrl.N1Max.Ki_array  InternalRulePriority=Speed
      settings: InputPortMap=u0,u1,u2,u3,u4,u5,u6,u7
  Kp Interpolation Using Prelookup : Interpolation_n-D  NumberOfTableDimensions=4  Table=MWS.Cntrl.WfCntrl.N1Max.Kp_array  InternalRulePriority=Speed
      settings: InputPortMap=u0,u1,u2,u3,u4,u5,u6,u7
  Sum : Sum  Inputs=|+-
  Sum1 : Sum  Inputs=|++
  Sum2 : Sum  Inputs=|-+
  Sum3 : Sum  Inputs=|+-
  Sum4 : Sum  Inputs=|++
  N1cDmd : Outport  VectorParamsAs1DForOutWhenUnconnected=off
  N1Max_SP : Outport  Port=2  VectorParamsAs1DForOutWhenUnconnected=off
  wires:
  N1/1 -> Sum/2
  Divide3/1 -> Sum1/1
  [Error] -> Divide3/2
  Sum1/1 -> Sum4/1
  Kp Interpolation Using Prelookup/1 -> Divide3/1  "Kp"
  [Error] -> Sum3/1
  Discrete-Time Integrator/1 -> Sum1/2
  Constant1/1 -> Sum/1, N1Max_SP/1  "N1_SP"
  Constant/1 -> Sum4/2
  Sum/1 -> [Error]
  Divide2/1 -> Discrete-Time Integrator/1
  Ki Interpolation Using Prelookup/1 -> Divide2/1  "Ki"
  Sum2/1 -> Gain/1
  N1cCmd/1 -> Sum2/1
  Gain/1 -> Sum3/2
  Sum4/1 -> Sum2/2, N1cDmd/1
  Sum3/1 -> Divide2/2
  Bus Selector/2 -> Ki Interpolation Using Prelookup/2, Kp Interpolation Using Prelookup/2  "<f_Alt>"
  Bus Selector/1 -> Ki Interpolation Using Prelookup/1, Kp Interpolation Using Prelookup/1  "<k_Alt>"
  Prelookup/1 -> Bus Selector/1
  Bus Selector/3 -> Ki Interpolation Using Prelookup/3, Kp Interpolation Using Prelookup/3  "<k_MN>"
  Bus Selector/4 -> Ki Interpolation Using Prelookup/4, Kp Interpolation Using Prelookup/4  "<f_MN>"
  Bus Selector/5 -> Ki Interpolation Using Prelookup/5, Kp Interpolation Using Prelookup/5  "<k_PwrInLP>"
  Bus Selector/6 -> Ki Interpolation Using Prelookup/6, Kp Interpolation Using Prelookup/6  "<f_PwrInLP>"
  Bus Selector/7 -> Ki Interpolation Using Prelookup/7, Kp Interpolation Using Prelookup/7  "<k_PwrInHP>"
  Bus Selector/8 -> Ki Interpolation Using Prelookup/8, Kp Interpolation Using Prelookup/8  "<f_PwrInHP>"

== system AGTF30SysDyn_PExPIn/Control System/Wf Controller/Controller/N1cSP Limit Controllers/N3 Max Controller ==
  Prelookup : Inport
  N3 : Inport  Port=2
  N1cCmd : Inport  Port=3
  Bus Selector : BusSelector  OutputSignals=k_Alt,f_Alt,k_MN,f_MN,k_PwrInLP,f_PwrInLP,k_PwrInHP,f_PwrInHP
  Constant : Constant  Value=MWS.Init.IC.N1c
  Constant1 : Constant  Value=MWS.Cntrl.WfCntrl.N3Max.SP
  Discrete-Time Integrator : DiscreteIntegrator  SampleTime=MWS.In.Ts  ICPrevOutput=DiscIntNeverNeededParam  ICPrevScaledInput=DiscIntNeverNeededParam
  Divide2 : Product  Inputs=**
  Divide3 : Product  Inputs=**
  Gain : Gain  Gain=MWS.Cntrl.WfCntrl.N3Max.Kiwp
  Ki Interpolation Using Prelookup : Interpolation_n-D  NumberOfTableDimensions=4  Table=MWS.Cntrl.WfCntrl.N3Max.Ki_array  InternalRulePriority=Speed
      settings: InputPortMap=u0,u1,u2,u3,u4,u5,u6,u7
  Kp Interpolation Using Prelookup : Interpolation_n-D  NumberOfTableDimensions=4  Table=MWS.Cntrl.WfCntrl.N3Max.Kp_array  InternalRulePriority=Speed
      settings: InputPortMap=u0,u1,u2,u3,u4,u5,u6,u7
  Sum : Sum  Inputs=|+-
  Sum1 : Sum  Inputs=|++
  Sum2 : Sum  Inputs=|-+
  Sum3 : Sum  Inputs=|+-
  Sum4 : Sum  Inputs=|++
  N1cDmd : Outport  VectorParamsAs1DForOutWhenUnconnected=off
  N3Max_SP : Outport  Port=2  VectorParamsAs1DForOutWhenUnconnected=off
  wires:
  Sum3/1 -> Divide2/2
  Ki Interpolation Using Prelookup/1 -> Divide2/1  "Ki"
  Divide2/1 -> Discrete-Time Integrator/1
  Sum/1 -> [Error]
  Constant/1 -> Sum4/2
  Constant1/1 -> N3Max_SP/1, Sum/1  "N3_SP"
  Discrete-Time Integrator/1 -> Sum1/2
  [Error] -> Sum3/1
  Kp Interpolation Using Prelookup/1 -> Divide3/1  "Kp"
  Sum1/1 -> Sum4/1
  [Error] -> Divide3/2
  Divide3/1 -> Sum1/1
  N3/1 -> Sum/2
  Sum4/1 -> Sum2/2, N1cDmd/1
  Gain/1 -> Sum3/2
  N1cCmd/1 -> Sum2/1
  Sum2/1 -> Gain/1
  Bus Selector/2 -> Ki Interpolation Using Prelookup/2, Kp Interpolation Using Prelookup/2  "<f_Alt>"
  Bus Selector/1 -> Ki Interpolation Using Prelookup/1, Kp Interpolation Using Prelookup/1  "<k_Alt>"
  Prelookup/1 -> Bus Selector/1
  Bus Selector/3 -> Ki Interpolation Using Prelookup/3, Kp Interpolation Using Prelookup/3  "<k_MN>"
  Bus Selector/4 -> Ki Interpolation Using Prelookup/4, Kp Interpolation Using Prelookup/4  "<f_MN>"
  Bus Selector/5 -> Ki Interpolation Using Prelookup/5, Kp Interpolation Using Prelookup/5  "<k_PwrInLP>"
  Bus Selector/6 -> Ki Interpolation Using Prelookup/6, Kp Interpolation Using Prelookup/6  "<f_PwrInLP>"
  Bus Selector/7 -> Ki Interpolation Using Prelookup/7, Kp Interpolation Using Prelookup/7  "<k_PwrInHP>"
  Bus Selector/8 -> Ki Interpolation Using Prelookup/8, Kp Interpolation Using Prelookup/8  "<f_PwrInHP>"

== system AGTF30SysDyn_PExPIn/Control System/Wf Controller/Controller/N1cSP Limit Controllers/Ps3 Max Controller ==
  Prelookup : Inport
  Ps3 : Inport  Port=2
  N1cCmd : Inport  Port=3
  Bus Selector : BusSelector  OutputSignals=k_Alt,f_Alt,k_MN,f_MN,k_PwrInLP,f_PwrInLP,k_PwrInHP,f_PwrInHP
  Constant : Constant  Value=MWS.Init.IC.N1c
  Constant1 : Constant  Value=MWS.Cntrl.WfCntrl.Ps3Max.SP
  Discrete-Time Integrator : DiscreteIntegrator  SampleTime=MWS.In.Ts  ICPrevOutput=DiscIntNeverNeededParam  ICPrevScaledInput=DiscIntNeverNeededParam
  Divide2 : Product  Inputs=**
  Divide3 : Product  Inputs=**
  Gain : Gain  Gain=MWS.Cntrl.WfCntrl.Ps3Max.Kiwp
  Ki Interpolation Using Prelookup : Interpolation_n-D  NumberOfTableDimensions=4  Table=MWS.Cntrl.WfCntrl.Ps3Max.Ki_array  InternalRulePriority=Speed
      settings: InputPortMap=u0,u1,u2,u3,u4,u5,u6,u7
  Kp Interpolation Using Prelookup : Interpolation_n-D  NumberOfTableDimensions=4  Table=MWS.Cntrl.WfCntrl.Ps3Max.Kp_array  InternalRulePriority=Speed
      settings: InputPortMap=u0,u1,u2,u3,u4,u5,u6,u7
  Sum : Sum  Inputs=|+-
  Sum1 : Sum  Inputs=|++
  Sum2 : Sum  Inputs=|-+
  Sum3 : Sum  Inputs=|+-
  Sum4 : Sum  Inputs=|++
  N1cDmd : Outport  VectorParamsAs1DForOutWhenUnconnected=off
  Ps3Max_SP : Outport  Port=2  VectorParamsAs1DForOutWhenUnconnected=off
  wires:
  Divide3/1 -> Sum1/1
  [Error] -> Divide3/2
  Sum1/1 -> Sum4/1
  Kp Interpolation Using Prelookup/1 -> Divide3/1  "Kp"
  [Error] -> Sum3/1
  Discrete-Time Integrator/1 -> Sum1/2
  Constant/1 -> Sum4/2
  Divide2/1 -> Discrete-Time Integrator/1
  Ki Interpolation Using Prelookup/1 -> Divide2/1  "Ki"
  Ps3/1 -> Sum/2
  Constant1/1 -> Ps3Max_SP/1, Sum/1  "Ps3_SP"
  Sum/1 -> [Error]
  Sum2/1 -> Gain/1
  N1cCmd/1 -> Sum2/1
  Gain/1 -> Sum3/2
  Sum4/1 -> Sum2/2, N1cDmd/1
  Sum3/1 -> Divide2/2
  Bus Selector/2 -> Ki Interpolation Using Prelookup/2, Kp Interpolation Using Prelookup/2  "<f_Alt>"
  Bus Selector/1 -> Ki Interpolation Using Prelookup/1, Kp Interpolation Using Prelookup/1  "<k_Alt>"
  Prelookup/1 -> Bus Selector/1
  Bus Selector/3 -> Ki Interpolation Using Prelookup/3, Kp Interpolation Using Prelookup/3  "<k_MN>"
  Bus Selector/4 -> Ki Interpolation Using Prelookup/4, Kp Interpolation Using Prelookup/4  "<f_MN>"
  Bus Selector/5 -> Ki Interpolation Using Prelookup/5, Kp Interpolation Using Prelookup/5  "<k_PwrInLP>"
  Bus Selector/6 -> Ki Interpolation Using Prelookup/6, Kp Interpolation Using Prelookup/6  "<f_PwrInLP>"
  Bus Selector/7 -> Ki Interpolation Using Prelookup/7, Kp Interpolation Using Prelookup/7  "<k_PwrInHP>"
  Bus Selector/8 -> Ki Interpolation Using Prelookup/8, Kp Interpolation Using Prelookup/8  "<f_PwrInHP>"

== system AGTF30SysDyn_PExPIn/Control System/Wf Controller/Controller/N1cSP Limit Controllers/Ps3 Min Controller ==
  Prelookup : Inport
  Ps3 : Inport  Port=2
  N1cCmd : Inport  Port=3
  Bus Selector : BusSelector  OutputSignals=k_Alt,f_Alt,k_MN,f_MN,k_PwrInLP,f_PwrInLP,k_PwrInHP,f_PwrInHP,k_PwrInHP_Ps3Min,f_PwrInHP_Ps3Min
  Constant : Constant  Value=MWS.Init.IC.N1c
  Discrete-Time Integrator : DiscreteIntegrator  SampleTime=MWS.In.Ts  ICPrevOutput=DiscIntNeverNeededParam  ICPrevScaledInput=DiscIntNeverNeededParam
  Divide2 : Product  Inputs=**
  Divide3 : Product  Inputs=**
  Gain : Gain  Gain=MWS.Cntrl.WfCntrl.Ps3Min.Kiwp
  Ki Interpolation Using Prelookup : Interpolation_n-D  NumberOfTableDimensions=3  Table=MWS.Cntrl.WfCntrl.Ps3Min.Ki_array  InternalRulePriority=Speed
      settings: InputPortMap=u0,u1,u2,u3,u4,u5
  Kp Interpolation Using Prelookup : Interpolation_n-D  NumberOfTableDimensions=3  Table=MWS.Cntrl.WfCntrl.Ps3Min.Kp_array  InternalRulePriority=Speed
      settings: InputPortMap=u0,u1,u2,u3,u4,u5
  Ps3minSP Interpolation Using Prelookup : Interpolation_n-D  NumberOfTableDimensions=4  Table=MWS.Cntrl.WfCntrl.Sched.Ps3MinSP.Ps3MinSP_array  InternalRulePriority=Speed
      settings: InputPortMap=u0,u1,u2,u3,u4,u5,u6,u7
  Sum : Sum  Inputs=|+-
  Sum1 : Sum  Inputs=|++
  Sum2 : Sum  Inputs=|-+
  Sum3 : Sum  Inputs=|+-
  Sum4 : Sum  Inputs=|++
  N1cDmd : Outport  VectorParamsAs1DForOutWhenUnconnected=off
  Ps3Min_SP : Outport  Port=2  VectorParamsAs1DForOutWhenUnconnected=off
  wires:
  Sum3/1 -> Divide2/2
  Ki Interpolation Using Prelookup/1 -> Divide2/1  "Ki"
  Divide2/1 -> Discrete-Time Integrator/1
  Sum/1 -> [Error]
  Constant/1 -> Sum4/2
  Ps3minSP Interpolation Using Prelookup/1 -> Ps3Min_SP/1, Sum/1  "Ps3min_SP"
  Discrete-Time Integrator/1 -> Sum1/2
  [Error] -> Sum3/1
  Kp Interpolation Using Prelookup/1 -> Divide3/1  "Kp"
  Sum1/1 -> Sum4/1
  [Error] -> Divide3/2
  Divide3/1 -> Sum1/1
  Ps3/1 -> Sum/2
  Sum4/1 -> Sum2/2, N1cDmd/1
  Sum2/1 -> Gain/1
  N1cCmd/1 -> Sum2/1
  Gain/1 -> Sum3/2
  Bus Selector/5 -> Ps3minSP Interpolation Using Prelookup/5  "<k_PwrInLP>"
  Bus Selector/2 -> Ki Interpolation Using Prelookup/2, Kp Interpolation Using Prelookup/2, Ps3minSP Interpolation Using Prelookup/2  "<f_Alt>"
  Bus Selector/1 -> Ps3minSP Interpolation Using Prelookup/1, Ki Interpolation Using Prelookup/1, Kp Interpolation Using Prelookup/1  "<k_Alt>"
  Bus Selector/6 -> Ps3minSP Interpolation Using Prelookup/6  "<f_PwrInLP>"
  Prelookup/1 -> Bus Selector/1
  Bus Selector/3 -> Ki Interpolation Using Prelookup/3, Kp Interpolation Using Prelookup/3, Ps3minSP Interpolation Using Prelookup/3  "<k_MN>"
  Bus Selector/4 -> Ki Interpolation Using Prelookup/4, Kp Interpolation Using Prelookup/4, Ps3minSP Interpolation Using Prelookup/4  "<f_MN>"
  Bus Selector/7 -> Ps3minSP Interpolation Using Prelookup/7  "<k_PwrInHP>"
  Bus Selector/8 -> Ps3minSP Interpolation Using Prelookup/8  "<f_PwrInHP>"
  Bus Selector/9 -> Ki Interpolation Using Prelookup/5, Kp Interpolation Using Prelookup/5  "<k_PwrInHP_Ps3Min>"
  Bus Selector/10 -> Ki Interpolation Using Prelookup/6, Kp Interpolation Using Prelookup/6  "<f_PwrInHP_Ps3Min>"

== system AGTF30SysDyn_PExPIn/Control System/Wf Controller/Controller/N1cSP Limit Controllers/T3 Max Controller ==
  Prelookup : Inport
  T3 : Inport  Port=2
  N1cCmd : Inport  Port=3
  Bus Selector : BusSelector  OutputSignals=k_Alt,f_Alt,k_MN,f_MN,k_PwrInLP,f_PwrInLP,k_PwrInHP,f_PwrInHP
  Constant : Constant  Value=MWS.Init.IC.N1c
  Constant1 : Constant  Value=MWS.Cntrl.WfCntrl.T3Max.SP
  Discrete-Time Integrator : DiscreteIntegrator  SampleTime=MWS.In.Ts  ICPrevOutput=DiscIntNeverNeededParam  ICPrevScaledInput=DiscIntNeverNeededParam
  Divide2 : Product  Inputs=**
  Divide3 : Product  Inputs=**
  Gain : Gain  Gain=MWS.Cntrl.WfCntrl.T3Max.Kiwp
  Ki Interpolation Using Prelookup : Interpolation_n-D  NumberOfTableDimensions=4  Table=MWS.Cntrl.WfCntrl.T3Max.Ki_array  InternalRulePriority=Speed
      settings: InputPortMap=u0,u1,u2,u3,u4,u5,u6,u7
  Kp Interpolation Using Prelookup : Interpolation_n-D  NumberOfTableDimensions=4  Table=MWS.Cntrl.WfCntrl.T3Max.Kp_array  InternalRulePriority=Speed
      settings: InputPortMap=u0,u1,u2,u3,u4,u5,u6,u7
  Sum : Sum  Inputs=|+-
  Sum1 : Sum  Inputs=|++
  Sum2 : Sum  Inputs=|-+
  Sum3 : Sum  Inputs=|+-
  Sum4 : Sum  Inputs=|++
  N1cDmd : Outport  VectorParamsAs1DForOutWhenUnconnected=off
  T3Max_SP : Outport  Port=2  VectorParamsAs1DForOutWhenUnconnected=off
  wires:
  Divide3/1 -> Sum1/1
  [Error] -> Divide3/2
  Sum1/1 -> Sum4/1
  Sum4/1 -> Sum2/2, N1cDmd/1
  Kp Interpolation Using Prelookup/1 -> Divide3/1  "Kp"
  [Error] -> Sum3/1
  Discrete-Time Integrator/1 -> Sum1/2
  Constant/1 -> Sum4/2
  Divide2/1 -> Discrete-Time Integrator/1
  Ki Interpolation Using Prelookup/1 -> Divide2/1  "Ki"
  Sum3/1 -> Divide2/2
  T3/1 -> Sum/2
  Constant1/1 -> T3Max_SP/1, Sum/1  "T3_SP"
  Sum/1 -> [Error]
  N1cCmd/1 -> Sum2/1
  Sum2/1 -> Gain/1
  Gain/1 -> Sum3/2
  Prelookup/1 -> Bus Selector/1
  Bus Selector/1 -> Ki Interpolation Using Prelookup/1, Kp Interpolation Using Prelookup/1  "<k_Alt>"
  Bus Selector/2 -> Ki Interpolation Using Prelookup/2, Kp Interpolation Using Prelookup/2  "<f_Alt>"
  Bus Selector/3 -> Ki Interpolation Using Prelookup/3, Kp Interpolation Using Prelookup/3  "<k_MN>"
  Bus Selector/4 -> Ki Interpolation Using Prelookup/4, Kp Interpolation Using Prelookup/4  "<f_MN>"
  Bus Selector/5 -> Ki Interpolation Using Prelookup/5, Kp Interpolation Using Prelookup/5  "<k_PwrInLP>"
  Bus Selector/6 -> Ki Interpolation Using Prelookup/6, Kp Interpolation Using Prelookup/6  "<f_PwrInLP>"
  Bus Selector/7 -> Ki Interpolation Using Prelookup/7, Kp Interpolation Using Prelookup/7  "<k_PwrInHP>"
  Bus Selector/8 -> Ki Interpolation Using Prelookup/8, Kp Interpolation Using Prelookup/8  "<f_PwrInHP>"

== system AGTF30SysDyn_PExPIn/Control System/Wf Controller/Controller/N1cSP Limit Controllers/T4 Max Controller ==
  Prelookup : Inport
  T4 : Inport  Port=2
  N1cCmd : Inport  Port=3
  Bus Selector : BusSelector  OutputSignals=k_Alt,f_Alt,k_MN,f_MN,k_PwrInLP,f_PwrInLP,k_PwrInHP,f_PwrInHP
  Constant : Constant  Value=MWS.Init.IC.N1c
  Constant7 : Constant  Value=MWS.Cntrl.WfCntrl.T4Max.SP
  Discrete-Time Integrator : DiscreteIntegrator  SampleTime=MWS.In.Ts  ICPrevOutput=DiscIntNeverNeededParam  ICPrevScaledInput=DiscIntNeverNeededParam
  Divide2 : Product  Inputs=**
  Divide3 : Product  Inputs=**
  Gain : Gain  Gain=MWS.Cntrl.WfCntrl.T4Max.Kiwp
  Ki Interpolation Using Prelookup : Interpolation_n-D  NumberOfTableDimensions=4  Table=MWS.Cntrl.WfCntrl.T4Max.Ki_array  InternalRulePriority=Speed
      settings: InputPortMap=u0,u1,u2,u3,u4,u5,u6,u7
  Kp Interpolation Using Prelookup : Interpolation_n-D  NumberOfTableDimensions=4  Table=MWS.Cntrl.WfCntrl.T4Max.Kp_array  InternalRulePriority=Speed
      settings: InputPortMap=u0,u1,u2,u3,u4,u5,u6,u7
  Sum : Sum  Inputs=|+-
  Sum1 : Sum  Inputs=|++
  Sum2 : Sum  Inputs=|-+
  Sum3 : Sum  Inputs=|+-
  Sum4 : Sum  Inputs=|++
  N1cDmd : Outport  VectorParamsAs1DForOutWhenUnconnected=off
  T4Max_SP : Outport  Port=2  VectorParamsAs1DForOutWhenUnconnected=off
  wires:
  Ki Interpolation Using Prelookup/1 -> Divide2/1  "Ki"
  Divide2/1 -> Discrete-Time Integrator/1
  Sum/1 -> [Error]
  Constant/1 -> Sum4/2
  Constant7/1 -> Sum/1, T4Max_SP/1  "T4_SP"
  Discrete-Time Integrator/1 -> Sum1/2
  [Error] -> Sum3/1
  Kp Interpolation Using Prelookup/1 -> Divide3/1  "Kp"
  Sum1/1 -> Sum4/1
  [Error] -> Divide3/2
  Divide3/1 -> Sum1/1
  T4/1 -> Sum/2
  Sum2/1 -> Gain/1
  N1cCmd/1 -> Sum2/1
  Gain/1 -> Sum3/2
  Sum4/1 -> Sum2/2, N1cDmd/1
  Sum3/1 -> Divide2/2
  Prelookup/1 -> Bus Selector/1
  Bus Selector/2 -> Ki Interpolation Using Prelookup/2, Kp Interpolation Using Prelookup/2  "<f_Alt>"
  Bus Selector/1 -> Ki Interpolation Using Prelookup/1, Kp Interpolation Using Prelookup/1  "<k_Alt>"
  Bus Selector/3 -> Ki Interpolation Using Prelookup/3, Kp Interpolation Using Prelookup/3  "<k_MN>"
  Bus Selector/4 -> Ki Interpolation Using Prelookup/4, Kp Interpolation Using Prelookup/4  "<f_MN>"
  Bus Selector/5 -> Ki Interpolation Using Prelookup/5, Kp Interpolation Using Prelookup/5  "<k_PwrInLP>"
  Bus Selector/6 -> Ki Interpolation Using Prelookup/6, Kp Interpolation Using Prelookup/6  "<f_PwrInLP>"
  Bus Selector/7 -> Ki Interpolation Using Prelookup/7, Kp Interpolation Using Prelookup/7  "<k_PwrInHP>"
  Bus Selector/8 -> Ki Interpolation Using Prelookup/8, Kp Interpolation Using Prelookup/8  "<f_PwrInHP>"

== system AGTF30SysDyn_PExPIn/Control System/Wf Controller/Controller/N1cSP Limit Controllers/T45 Max Controller ==
  Prelookup : Inport
  T45 : Inport  Port=2
  N1cCmd : Inport  Port=3
  Bus Selector : BusSelector  OutputSignals=k_Alt,f_Alt,k_MN,f_MN,k_PwrInLP,f_PwrInLP,k_PwrInHP,f_PwrInHP
  Constant : Constant  Value=MWS.Init.IC.N1c
  Discrete-Time Integrator : DiscreteIntegrator  SampleTime=MWS.In.Ts  ICPrevOutput=DiscIntNeverNeededParam  ICPrevScaledInput=DiscIntNeverNeededParam
  Divide2 : Product  Inputs=**
  Divide3 : Product  Inputs=**
  Gain : Gain  Gain=MWS.Cntrl.WfCntrl.T45Max.Kiwp
  Ki Interpolation Using Prelookup : Interpolation_n-D  NumberOfTableDimensions=4  Table=MWS.Cntrl.WfCntrl.T45Max.Ki_array  InternalRulePriority=Speed
      settings: InputPortMap=u0,u1,u2,u3,u4,u5,u6,u7
  Kp Interpolation Using Prelookup : Interpolation_n-D  NumberOfTableDimensions=4  Table=MWS.Cntrl.WfCntrl.T45Max.Kp_array  InternalRulePriority=Speed
      settings: InputPortMap=u0,u1,u2,u3,u4,u5,u6,u7
  Sum : Sum  Inputs=|+-
  Sum1 : Sum  Inputs=|++
  Sum2 : Sum  Inputs=|-+
  Sum3 : Sum  Inputs=|+-
  Sum4 : Sum  Inputs=|++
  T45 Max Set-Point Interpolation Using Prelookup : Interpolation_n-D  NumberOfTableDimensions=4  Table=MWS.Cntrl.WfCntrl.Sched.T45MaxSP.T45MaxSP_array  InternalRulePriority=Speed
      settings: InputPortMap=u0,u1,u2,u3,u4,u5,u6,u7
  N1cDmd : Outport  VectorParamsAs1DForOutWhenUnconnected=off
  T4Max_SP : Outport  Port=2  VectorParamsAs1DForOutWhenUnconnected=off
  wires:
  Prelookup/1 -> Bus Selector/1
  Sum3/1 -> Divide2/2
  Sum4/1 -> N1cDmd/1, Sum2/2
  Gain/1 -> Sum3/2
  N1cCmd/1 -> Sum2/1
  Sum2/1 -> Gain/1
  T45/1 -> Sum/2
  Divide3/1 -> Sum1/1
  [Error] -> Divide3/2
  Sum1/1 -> Sum4/1
  Kp Interpolation Using Prelookup/1 -> Divide3/1  "Kp"
  [Error] -> Sum3/1
  Discrete-Time Integrator/1 -> Sum1/2
  T45 Max Set-Point Interpolation Using Prelookup/1 -> Sum/1, T4Max_SP/1  "T5_SP"
  Constant/1 -> Sum4/2
  Sum/1 -> [Error]
  Divide2/1 -> Discrete-Time Integrator/1
  Ki Interpolation Using Prelookup/1 -> Divide2/1  "Ki"
  Bus Selector/1 -> Ki Interpolation Using Prelookup/1, Kp Interpolation Using Prelookup/1, T45 Max Set-Point Interpolation Using Prelookup/1  "<k_Alt>"
  Bus Selector/2 -> Ki Interpolation Using Prelookup/2, Kp Interpolation Using Prelookup/2, T45 Max Set-Point Interpolation Using Prelookup/2  "<f_Alt>"
  Bus Selector/3 -> Kp Interpolation Using Prelookup/3, Ki Interpolation Using Prelookup/3, T45 Max Set-Point Interpolation Using Prelookup/3  "<k_MN>"
  Bus Selector/4 -> Kp Interpolation Using Prelookup/4, Ki Interpolation Using Prelookup/4, T45 Max Set-Point Interpolation Using Prelookup/4  "<f_MN>"
  Bus Selector/5 -> Ki Interpolation Using Prelookup/5, Kp Interpolation Using Prelookup/5, T45 Max Set-Point Interpolation Using Prelookup/5  "<k_PwrInLP>"
  Bus Selector/6 -> Ki Interpolation Using Prelookup/6, Kp Interpolation Using Prelookup/6, T45 Max Set-Point Interpolation Using Prelookup/6  "<f_PwrInLP>"
  Bus Selector/7 -> Ki Interpolation Using Prelookup/7, Kp Interpolation Using Prelookup/7, T45 Max Set-Point Interpolation Using Prelookup/7  "<k_PwrInHP>"
  Bus Selector/8 -> Ki Interpolation Using Prelookup/8, Kp Interpolation Using Prelookup/8, T45 Max Set-Point Interpolation Using Prelookup/8  "<f_PwrInHP>"
